simulink model "problem3b_translation_system"  (R2024b)
settings: Solver=ode45  StartTime=0.0  StopTime=Sim_Time  MaxStep=0.01  RelTol=1e-3  EnableMultiTasking=on
undefined symbols (not defined in the file): F
settings Model: Creator=dzr3qn  LastModifiedBy=karltzu
settings SolverCC: AlgebraicLoopSolver=TrustRegion
settings DataIOCC: LimitDataPoints=on  SaveFormat=Array  ReturnWorkspaceOutputs=off
settings OptimizationCC: LifeSpan=inf
settings DebuggingCC: SolverPrmCheckMsg=warning  UnconnectedInputMsg=warning  UnconnectedOutputMsg=warning  UnconnectedLineMsg=warning  SFUnexpectedBacktrackingDiag=warning  SFNoUnconditionalDefaultTransitionDiag=warning  SFExecutionAtInitializationDiag=none  ArithmeticOperatorsInVariantConditions=warning
settings HardwareCC: ProdBitPerPointer=32  ProdBitPerSizeT=32  ProdBitPerPtrDiffT=32  ProdLargestAtomicFloat=None  ProdIntDivRoundTo=Undefined  ProdEndianess=Unspecified  ProdWordSize=32  ProdHWDeviceType=32-bit Generic
settings ModelReferenceCC: EnableRefExpFcnMdlSchedulingChecks=on  PropagateSignalLabelsOutOfModel=off
settings SFSimCC: SimUseLocalCustomCode=off  CustomCodeUndefinedFunction=UseInterfaceOnly
settings RTWCC: RTWUseLocalCustomCode=off  GPUComputeCapability=3.5
settings CodeAppCC: StateflowObjectComments=on
settings GRTTargetCC: TargetLangStandard=C89/C90 (ANSI)
settings ConfigComp: CovMetricSettings=dw  CovSaveCumulativeToWorkspaceVar=on  CovSaveSingleToWorkspaceVar=on  CovExternalEMLEnable=off  CovSFcnEnable=off

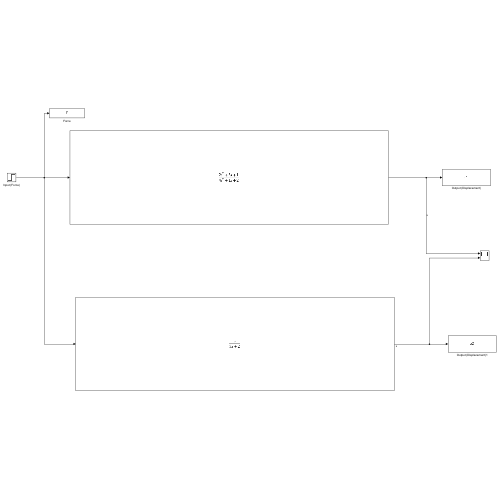
[thumbnail: Simulink's stored preview of the top-level diagram]
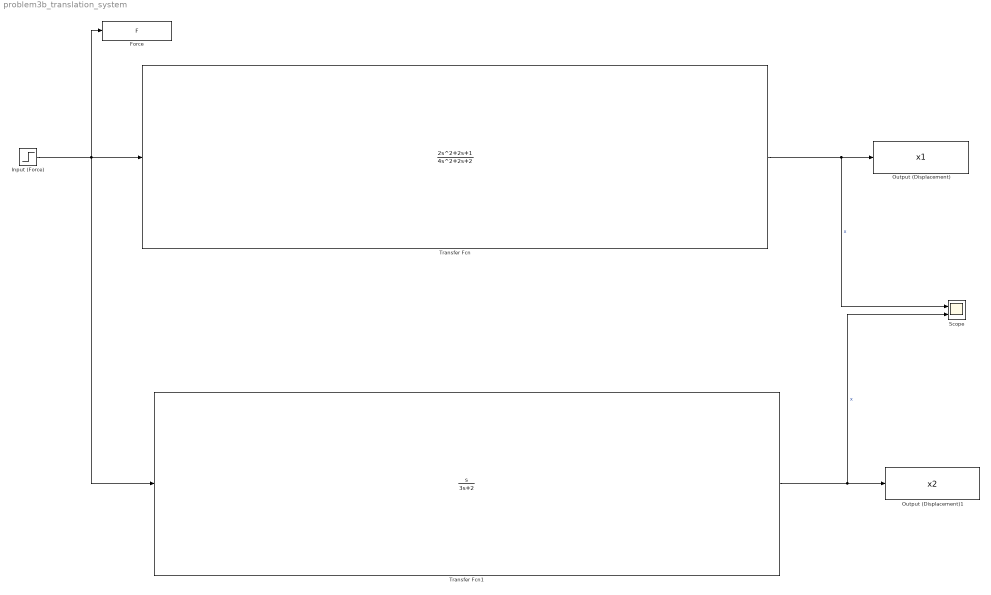
== system problem3b_translation_system ==
  Force : ToWorkspace  VariableName=F  SaveFormat=Timeseries  SampleTime=-1
  Input (Force) : Step  After=F  SampleTime=0  ZeroCross=off
  Output (Displacement) : ToWorkspace  VariableName=x1  SaveFormat=Timeseries  SampleTime=-1
  Output (Displacement)1 : ToWorkspace  VariableName=x2  SaveFormat=Timeseries  SampleTime=-1
  Scope : Scope  NumInputPorts=2
  Transfer Fcn : TransferFcn  Numerator=[2 2 1]  Denominator=[4 2 2]
  Transfer Fcn1 : TransferFcn  Numerator=[1 0]  Denominator=[0 3 2]
  wires:
  Input (Force)/1 -> Transfer Fcn1/1, Transfer Fcn/1, Force/1
  Transfer Fcn/1 -> Scope/1, Output (Displacement)/1  "x"
  Transfer Fcn1/1 -> Scope/2, Output (Displacement)1/1  "x"
